simulink model "modele_gyros_BF1"  (Simulink 8.3)
settings: Solver=ode45  StartTime=0.0  StopTime=t_sim  RelTol=1e-3
values from neighbouring files (symbols this model uses):
  A = [0   0   0   0   1   0   0   0 ... (first row only)    [state_model_data.m]
  B = [0   0   0   0 ... (first row only)    [state_model_data.m]
  C = eye(8)    [state_model_data.m]
  Choix = 3    [script_axe3_BF.m]
  D = zeros(8, 4)    [state_model_data.m]
  Kg = 1/2*wn/zeta    (= 10.7142857143)    [script_axe3_BF.m]
  Kpv = 2*(Ic+Id)*wn*zeta    [script_axe3_BF.m]
  Omega1_0 = Omega1_c*2*pi/60    (= 41.8879020479)    [script_axe3_BF.m]
  Omega1_c = 400    [script_axe3_BF.m]
  Omega2_0 = 0    [script_axe3_BF.m]
  q20 = -pi/2    (= -1.57079632679)    [Traces_Gyros.m]    (also in script_axe3_BF.m = 0; state_model_data.m = 0)
  q30 = -pi/2    (= -1.57079632679)    [Traces_Gyros.m]    (also in script_axe3_BF.m = 0; state_model_data.m = 0)
undefined symbols (not defined in the file or in its folder): K1, K2, K3, K4, Kamp, Km1, Km2, Kv2, Kv3, Kv4, Omega2_c, Omega3_c, Omega4_c
libraries: library_gyro x1
settings Model: Creator=ahmed.chaibet  LastModifiedBy=ahmed.chaibet
settings OptimizationCC: ExpressionDepthLimit=2147483647
settings DebuggingCC: SaveWithParameterizedLinksMsg=none  SignalResolutionControl=TryResolveAllWithWarning  SolverPrmCheckMsg=none  MultiTaskDSMMsg=warning  MultiTaskCondExecSysMsg=none  StrictBusMsg=None
settings HardwareCC: TargetUnknown=on
settings RTWCC: IncludeERTFirstTime=on

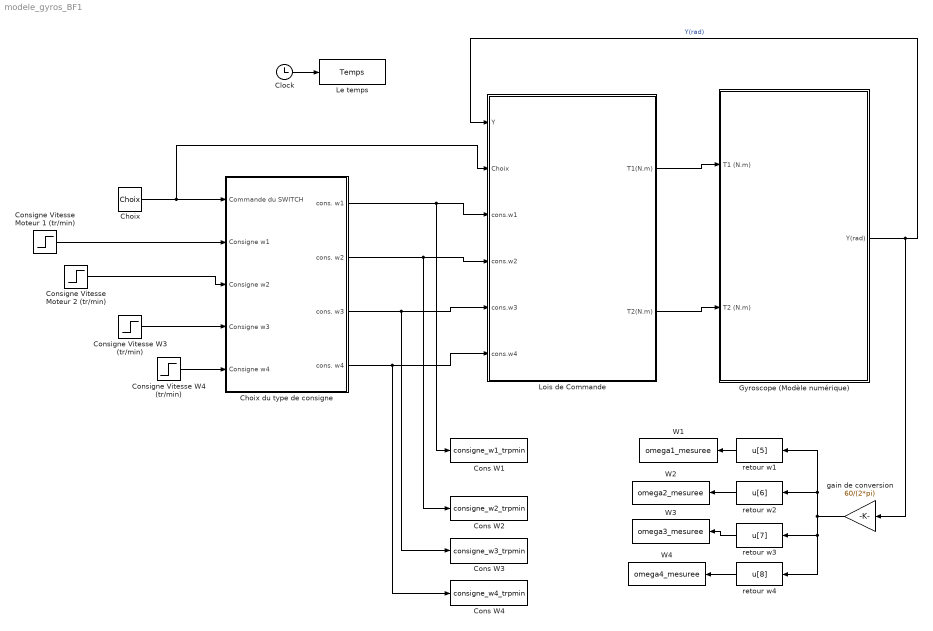
== system modele_gyros_BF1 ==
  Choix : Constant  Value=Choix
  Choix du type de consigne : Subsystem
  Clock : Clock
  Cons W1 : ToWorkspace  VariableName=consigne_w1_trpmin  SampleTime=-1
  Cons W2 : ToWorkspace  VariableName=consigne_w2_trpmin  SampleTime=-1
  Cons W3 : ToWorkspace  VariableName=consigne_w3_trpmin  SampleTime=-1
  Cons W4 : ToWorkspace  VariableName=consigne_w4_trpmin  SampleTime=-1
  Consigne Vitesse Moteur 1 (tr/min) : Step  Time=0  After=Omega1_c  SampleTime=0
  Consigne Vitesse Moteur 2 (tr/min) : Step  Time=0  After=Omega2_c  SampleTime=0
  Consigne Vitesse W3 (tr/min) : Step  Time=0  After=Omega3_c  SampleTime=0
  Consigne Vitesse W4 (tr/min) : Step  Time=0  After=Omega4_c  SampleTime=0
  Gyroscope (Modèle numérique) : Subsystem
  Le temps : ToWorkspace  VariableName=Temps  SampleTime=-1
  Lois de Commande : Subsystem
  W1 : ToWorkspace  VariableName=omega1_mesuree  SampleTime=-1
  W2 : ToWorkspace  VariableName=omega2_mesuree  SampleTime=-1
  W3 : ToWorkspace  VariableName=omega3_mesuree  SampleTime=-1
  W4 : ToWorkspace  VariableName=omega4_mesuree  SampleTime=-1
  gain de conversion : Gain  Gain=60/(2*pi)  SaturateOnIntegerOverflow=on  OutDataTypeStr=Inherit: Same as input  ParamDataTypeStr=Inherit: Same as input
  retour w1 : Fcn  Expr=u[5]
  retour w2 : Fcn  Expr=u[6]
  retour w3 : Fcn  Expr=u[7]
  retour w4 : Fcn  Expr=u[8]
  wires:
  Clock/1 -> Le temps/1
  Consigne Vitesse Moteur 1 (tr/min)/1 -> Choix du type de consigne/2(Consigne w1)
  Consigne Vitesse Moteur 2 (tr/min)/1 -> Choix du type de consigne/3(Consigne w2)
  Consigne Vitesse W3 (tr/min)/1 -> Choix du type de consigne/4(Consigne w3)
  Choix du type de consigne/1(cons. w1) -> Cons W1/1, Lois de Commande/3(cons.w1)
  Choix du type de consigne/2(cons. w2) -> Cons W2/1, Lois de Commande/4(cons.w2)
  Choix du type de consigne/3(cons. w3) -> Cons W3/1, Lois de Commande/5(cons.w3)
  Choix du type de consigne/4(cons. w4) -> Cons W4/1, Lois de Commande/6(cons.w4)
  Choix/1 -> Lois de Commande/2(Choix), Choix du type de consigne/1(Commande du SWITCH)
  Lois de Commande/1(T1(N.m)) -> Gyroscope (Modèle numérique)/1(T1 (N.m))
  Lois de Commande/2(T2(N.m)) -> Gyroscope (Modèle numérique)/2(T2 (N.m))
  Consigne Vitesse W4 (tr/min)/1 -> Choix du type de consigne/5(Consigne w4)
  Gyroscope (Modèle numérique)/1(Y(rad)) -> gain de conversion/1, Lois de Commande/1(Y)  "Y(rad)"
  gain de conversion/1 -> retour w1/1, retour w2/1, retour w4/1, retour w3/1
  retour w1/1 -> W1/1
  retour w2/1 -> W2/1
  retour w3/1 -> W3/1
  retour w4/1 -> W4/1

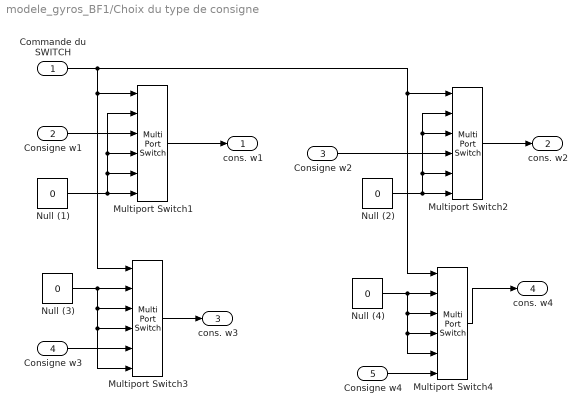
== system modele_gyros_BF1/Choix du type de consigne ==
  Commande du SWITCH : Inport
  Consigne w1 : Inport  Port=2
  Consigne w2 : Inport  Port=3
  Consigne w3 : Inport  Port=4
  Consigne w4 : Inport  Port=5
  Multiport Switch1 : MultiPortSwitch  Inputs=5  SaturateOnIntegerOverflow=on  InputSameDT=on
  Multiport Switch2 : MultiPortSwitch  Inputs=5  SaturateOnIntegerOverflow=on  InputSameDT=on
  Multiport Switch3 : MultiPortSwitch  Inputs=5  SaturateOnIntegerOverflow=on  InputSameDT=on
  "Multiport Switch4 " : MultiPortSwitch  Inputs=5  SaturateOnIntegerOverflow=on  InputSameDT=on
  Null (1) : Constant  Value=0
  Null (2) : Constant  Value=0
  Null (3) : Constant  Value=0
  Null (4) : Constant  Value=0
  cons. w1 : Outport
  cons. w2 : Outport  Port=2
  cons. w3 : Outport  Port=3
  cons. w4 : Outport  Port=4
  wires:
  Multiport Switch1/1 -> cons. w1/1
  Multiport Switch3/1 -> cons. w3/1
  Multiport Switch2/1 -> cons. w2/1
  "Multiport Switch4 "/1 -> cons. w4/1
  Commande du SWITCH/1 -> Multiport Switch1/1, Multiport Switch3/1, Multiport Switch2/1, "Multiport Switch4 "/1
  Consigne w1/1 -> Multiport Switch1/3
  Consigne w2/1 -> Multiport Switch2/4
  Consigne w3/1 -> Multiport Switch3/5
  Consigne w4/1 -> "Multiport Switch4 "/6
  Null (1)/1 -> Multiport Switch1/6, Multiport Switch1/5, Multiport Switch1/4, Multiport Switch1/2
  Null (2)/1 -> Multiport Switch2/6, Multiport Switch2/2, Multiport Switch2/3, Multiport Switch2/5
  Null (3)/1 -> Multiport Switch3/2, Multiport Switch3/3, Multiport Switch3/4, Multiport Switch3/6
  Null (4)/1 -> "Multiport Switch4 "/2, "Multiport Switch4 "/3, "Multiport Switch4 "/4, "Multiport Switch4 "/5

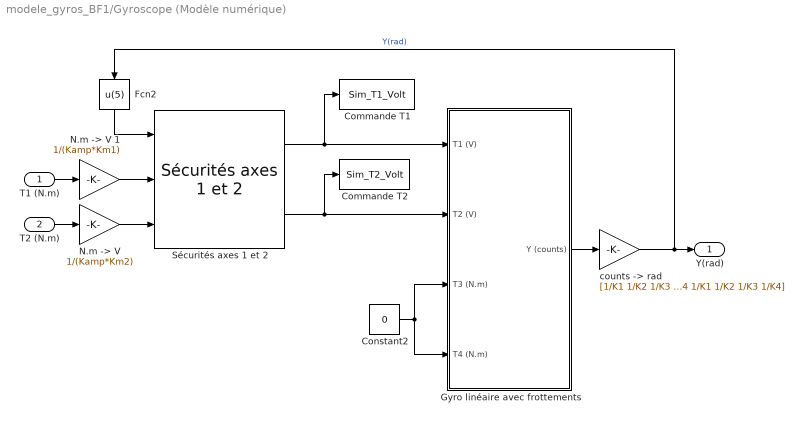
== system modele_gyros_BF1/Gyroscope (Modèle numérique) ==
  T1 (N.m) : Inport
  T2 (N.m) : Inport  Port=2
  Commande T1 : ToWorkspace  VariableName=Sim_T1_Volt  SampleTime=-1
  Commande T2 : ToWorkspace  VariableName=Sim_T2_Volt  SampleTime=-1
  Constant2 : Constant  Value=0
  Fcn2 : Fcn  Expr=u(5)
  Gyro linéaire avec frottements : Subsystem
  "N.m -> V" : Gain  Gain=1/(Kamp*Km2)  SaturateOnIntegerOverflow=on  OutDataTypeStr=Inherit: Same as input  ParamDataTypeStr=Inherit: Same as input
  "N.m -> V 1" : Gain  Gain=1/(Kamp*Km1)  SaturateOnIntegerOverflow=on  OutDataTypeStr=Inherit: Same as input  ParamDataTypeStr=Inherit: Same as input
  Sécurités axes 1 et 2 : library_gyro/Sécurités axes 1 et 2
  "counts -> rad" : Gain  Gain=[1/K1 1/K2 1/K3 1/K4 1/K1 1/K2 1/K3 1/K4]  SaturateOnIntegerOverflow=on  OutDataTypeStr=Inherit: Same as input  ParamDataTypeStr=Inherit: Same as input
  Y(rad) : Outport
  wires:
  Gyro linéaire avec frottements/1(Y (counts)) -> "counts -> rad"/1
  Sécurités axes 1 et 2/2 -> Gyro linéaire avec frottements/2(T2 (V)), Commande T2/1
  Sécurités axes 1 et 2/1 -> Gyro linéaire avec frottements/1(T1 (V)), Commande T1/1
  Constant2/1 -> Gyro linéaire avec frottements/4(T4 (N.m)), Gyro linéaire avec frottements/3(T3 (N.m))
  "N.m -> V"/1 -> Sécurités axes 1 et 2/3
  "counts -> rad"/1 -> Y(rad)/1, Fcn2/1  "Y(rad)"
  Fcn2/1 -> Sécurités axes 1 et 2/1
  "N.m -> V 1"/1 -> Sécurités axes 1 et 2/2
  T1 (N.m)/1 -> "N.m -> V 1"/1
  T2 (N.m)/1 -> "N.m -> V"/1

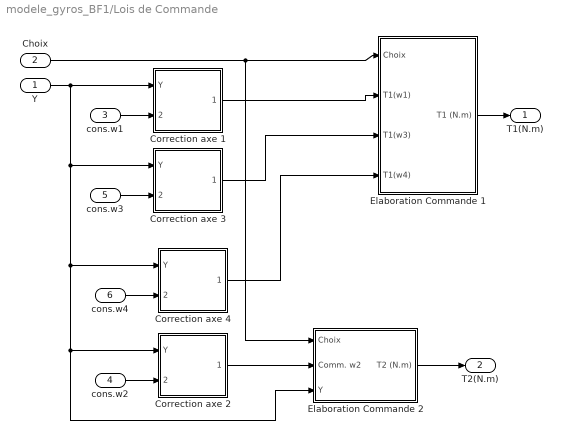
== system modele_gyros_BF1/Lois de Commande ==
  Y : Inport
  Choix : Inport  Port=2
  cons.w1 : Inport  Port=3
  cons.w2 : Inport  Port=4
  cons.w3 : Inport  Port=5
  cons.w4 : Inport  Port=6
  Correction axe 1 : Subsystem
  Correction axe 2 : Subsystem
  Correction axe 3 : Subsystem
  Correction axe 4 : Subsystem
  Elaboration Commande 1 : Subsystem
  Elaboration Commande 2 : Subsystem
  T1(N.m) : Outport
  T2(N.m) : Outport  Port=2
  wires:
  cons.w1/1 -> Correction axe 1/2(cons.w1)
  Correction axe 1/1(T1(w1)) -> Elaboration Commande 1/2(T1(w1))
  cons.w3/1 -> Correction axe 3/2(cons.w3)
  Correction axe 3/1(T1(w3)) -> Elaboration Commande 1/3(T1(w3))
  cons.w4/1 -> Correction axe 4/2(cons.w4)
  Correction axe 4/1(T2(w4)) -> Elaboration Commande 1/4(T1(w4))
  cons.w2/1 -> Correction axe 2/2(cons.w2)
  Correction axe 2/1(T2(w2)) -> Elaboration Commande 2/2(Comm. w2)
  Y/1 -> Correction axe 1/1(Y), Correction axe 3/1(Y), Correction axe 4/1(Y), Correction axe 2/1(Y), Elaboration Commande 2/3(Y)
  Elaboration Commande 1/1(T1 (N.m)) -> T1(N.m)/1
  Choix/1 -> Elaboration Commande 2/1(Choix), Elaboration Commande 1/1(Choix)
  Elaboration Commande 2/1(T2 (N.m)) -> T2(N.m)/1

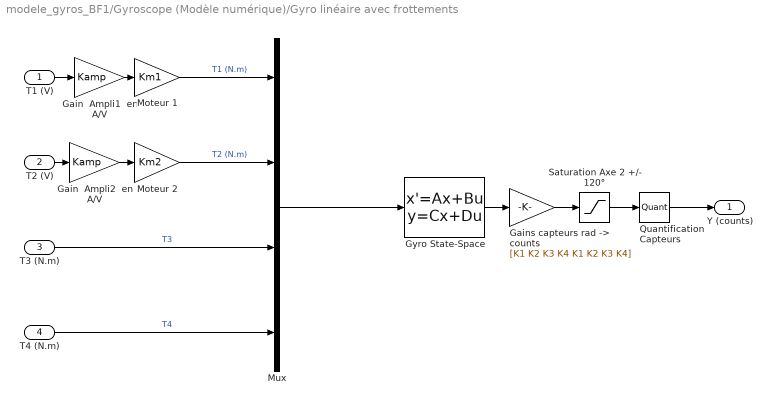
== system modele_gyros_BF1/Gyroscope (Modèle numérique)/Gyro linéaire avec frottements ==
  T1 (V) : Inport
  T2 (V) : Inport  Port=2
  T3 (N.m) : Inport  Port=3
  T4 (N.m) : Inport  Port=4
  Gain  Ampli1  en A/V : Gain  Gain=Kamp  SaturateOnIntegerOverflow=on  OutDataTypeStr=Inherit: Same as input  ParamDataTypeStr=Inherit: Same as input
  Gain  Ampli2  en A/V : Gain  Gain=Kamp  SaturateOnIntegerOverflow=on  OutDataTypeStr=Inherit: Same as input  ParamDataTypeStr=Inherit: Same as input
  "Gains capteurs rad -> counts" : Gain  Gain=[K1 K2 K3 K4 K1 K2 K3 K4]  SaturateOnIntegerOverflow=on  OutDataTypeStr=Inherit: Same as input  ParamDataTypeStr=Inherit: Same as input
  Gyro State-Space : StateSpace  A=A  B=B  C=C  D=D  X0=[0 q20 q30 0 Omega1_0 Omega2_0 0 0]
  Moteur 1 : Gain  Gain=Km1  SaturateOnIntegerOverflow=on  OutDataTypeStr=Inherit: Same as input  ParamDataTypeStr=Inherit: Same as input
  Moteur 2 : Gain  Gain=Km2  SaturateOnIntegerOverflow=on  OutDataTypeStr=Inherit: Same as input  ParamDataTypeStr=Inherit: Same as input
  Mux : Mux
  Quantification Capteurs : Quantizer  QuantizationInterval=Q
  Saturation Axe 2 +/- 120° : Saturate  UpperLimit=[inf 120*pi/180*K2 inf inf inf inf inf inf]  LowerLimit=[-inf -120*pi/180*K2 -inf -inf -inf -inf -inf -inf]
  Y (counts) : Outport
  wires:
  T1 (V)/1 -> Gain  Ampli1  en A/V/1
  Gain  Ampli1  en A/V/1 -> Moteur 1/1
  Moteur 2/1 -> Mux/2  "T2 (N.m)"
  Gain  Ampli2  en A/V/1 -> Moteur 2/1
  Gyro State-Space/1 -> "Gains capteurs rad -> counts"/1
  T2 (V)/1 -> Gain  Ampli2  en A/V/1
  Saturation Axe 2 +/- 120°/1 -> Quantification Capteurs/1
  Quantification Capteurs/1 -> Y (counts)/1
  T3 (N.m)/1 -> Mux/3  "T3"
  T4 (N.m)/1 -> Mux/4  "T4"
  "Gains capteurs rad -> counts"/1 -> Saturation Axe 2 +/- 120°/1
  Moteur 1/1 -> Mux/1  "T1 (N.m)"
  Mux/1 -> Gyro State-Space/1

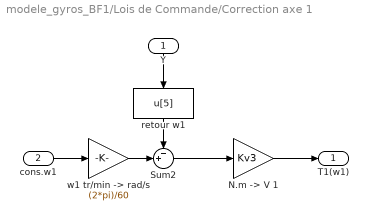
== system modele_gyros_BF1/Lois de Commande/Correction axe 1 ==
  Y : Inport
  cons.w1 : Inport  Port=2
  "N.m -> V 1" : Gain  Gain=Kv3  SaturateOnIntegerOverflow=on  OutDataTypeStr=Inherit: Same as input  ParamDataTypeStr=Inherit: Same as input
  Sum2 : Sum  Inputs=-+|  SaturateOnIntegerOverflow=on  InputSameDT=on  OutDataTypeStr=Inherit: Same as first input
  retour w1 : Fcn  Expr=u[5]
  "w1 tr/min -> rad/s" : Gain  Gain=(2*pi)/60  SaturateOnIntegerOverflow=on  OutDataTypeStr=Inherit: Same as input  ParamDataTypeStr=Inherit: Same as input
  T1(w1) : Outport
  wires:
  "w1 tr/min -> rad/s"/1 -> Sum2/2
  retour w1/1 -> Sum2/1
  Sum2/1 -> "N.m -> V 1"/1
  cons.w1/1 -> "w1 tr/min -> rad/s"/1
  "N.m -> V 1"/1 -> T1(w1)/1
  Y/1 -> retour w1/1

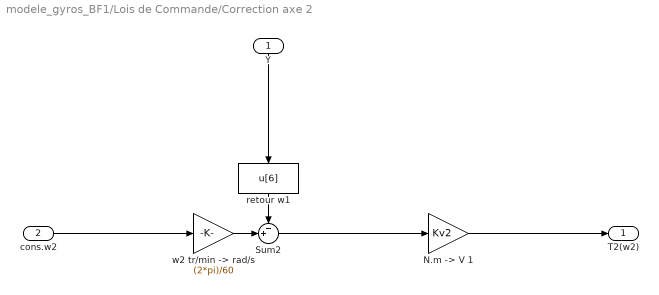
== system modele_gyros_BF1/Lois de Commande/Correction axe 2 ==
  Y : Inport
  cons.w2 : Inport  Port=2
  "N.m -> V 1" : Gain  Gain=Kv2  SaturateOnIntegerOverflow=on  OutDataTypeStr=Inherit: Same as input  ParamDataTypeStr=Inherit: Same as input
  Sum2 : Sum  Inputs=-+|  SaturateOnIntegerOverflow=on  InputSameDT=on  OutDataTypeStr=Inherit: Same as first input
  retour w1 : Fcn  Expr=u[6]
  "w2 tr/min -> rad/s" : Gain  Gain=(2*pi)/60  SaturateOnIntegerOverflow=on  OutDataTypeStr=Inherit: Same as input  ParamDataTypeStr=Inherit: Same as input
  T2(w2) : Outport
  wires:
  "w2 tr/min -> rad/s"/1 -> Sum2/2
  retour w1/1 -> Sum2/1
  Sum2/1 -> "N.m -> V 1"/1
  cons.w2/1 -> "w2 tr/min -> rad/s"/1
  "N.m -> V 1"/1 -> T2(w2)/1
  Y/1 -> retour w1/1

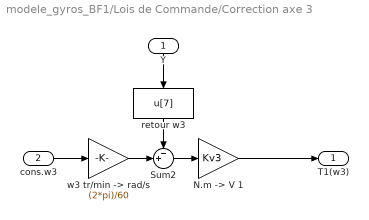
== system modele_gyros_BF1/Lois de Commande/Correction axe 3 ==
  Y : Inport
  cons.w3 : Inport  Port=2
  "N.m -> V 1" : Gain  Gain=Kv3  SaturateOnIntegerOverflow=on  OutDataTypeStr=Inherit: Same as input  ParamDataTypeStr=Inherit: Same as input
  Sum2 : Sum  Inputs=-+|  SaturateOnIntegerOverflow=on  InputSameDT=on  OutDataTypeStr=Inherit: Same as first input
  retour w3 : Fcn  Expr=u[7]
  "w3 tr/min -> rad/s" : Gain  Gain=(2*pi)/60  SaturateOnIntegerOverflow=on  OutDataTypeStr=Inherit: Same as input  ParamDataTypeStr=Inherit: Same as input
  T1(w3) : Outport
  wires:
  Y/1 -> retour w3/1
  "N.m -> V 1"/1 -> T1(w3)/1
  cons.w3/1 -> "w3 tr/min -> rad/s"/1
  Sum2/1 -> "N.m -> V 1"/1
  retour w3/1 -> Sum2/1
  "w3 tr/min -> rad/s"/1 -> Sum2/2

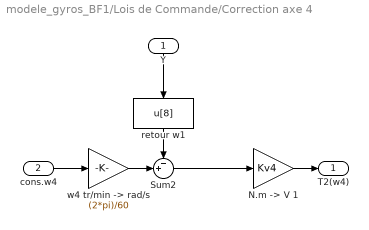
== system modele_gyros_BF1/Lois de Commande/Correction axe 4 ==
  Y : Inport
  cons.w4 : Inport  Port=2
  "N.m -> V 1" : Gain  Gain=Kv4  SaturateOnIntegerOverflow=on  OutDataTypeStr=Inherit: Same as input  ParamDataTypeStr=Inherit: Same as input
  Sum2 : Sum  Inputs=-+|  SaturateOnIntegerOverflow=on  InputSameDT=on  OutDataTypeStr=Inherit: Same as first input
  retour w1 : Fcn  Expr=u[8]
  "w4 tr/min -> rad/s" : Gain  Gain=(2*pi)/60  SaturateOnIntegerOverflow=on  OutDataTypeStr=Inherit: Same as input  ParamDataTypeStr=Inherit: Same as input
  T2(w4) : Outport
  wires:
  Y/1 -> retour w1/1
  "N.m -> V 1"/1 -> T2(w4)/1
  cons.w4/1 -> "w4 tr/min -> rad/s"/1
  Sum2/1 -> "N.m -> V 1"/1
  retour w1/1 -> Sum2/1
  "w4 tr/min -> rad/s"/1 -> Sum2/2

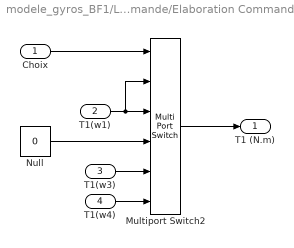
== system modele_gyros_BF1/Lois de Commande/Elaboration Commande 1 ==
  Choix : Inport
  T1(w1) : Inport  Port=2
  T1(w3) : Inport  Port=3
  T1(w4) : Inport  Port=4
  Multiport Switch2 : MultiPortSwitch  Inputs=5  SaturateOnIntegerOverflow=on  InputSameDT=on
  Null : Constant  Value=0
  T1 (N.m) : Outport
  wires:
  Choix/1 -> Multiport Switch2/1
  T1(w1)/1 -> Multiport Switch2/3, Multiport Switch2/2
  Multiport Switch2/1 -> T1 (N.m)/1
  T1(w3)/1 -> Multiport Switch2/5
  Null/1 -> Multiport Switch2/4
  T1(w4)/1 -> Multiport Switch2/6

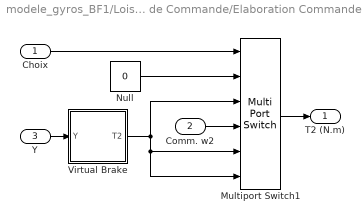
== system modele_gyros_BF1/Lois de Commande/Elaboration Commande 2 ==
  Choix : Inport
  Comm. w2 : Inport  Port=2
  Y : Inport  Port=3
  Multiport Switch1 : MultiPortSwitch  Inputs=5  SaturateOnIntegerOverflow=on  InputSameDT=on
  Null : Constant  Value=0
  Virtual Brake : Subsystem
  T2 (N.m) : Outport
  wires:
  Choix/1 -> Multiport Switch1/1
  Multiport Switch1/1 -> T2 (N.m)/1
  Y/1 -> Virtual Brake/1(Y)
  Null/1 -> Multiport Switch1/2
  Virtual Brake/1(T2) -> Multiport Switch1/3, Multiport Switch1/5, Multiport Switch1/6
  Comm. w2/1 -> Multiport Switch1/4

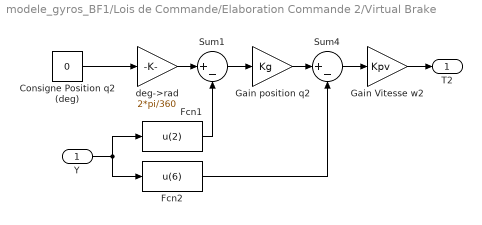
== system modele_gyros_BF1/Lois de Commande/Elaboration Commande 2/Virtual Brake ==
  Y : Inport
  Consigne Position q2 (deg) : Constant  Value=0
  Fcn1 : Fcn  Expr=u(2)
  Fcn2 : Fcn  Expr=u(6)
  Gain Vitesse w2 : Gain  Gain=Kpv  SaturateOnIntegerOverflow=on  OutDataTypeStr=Inherit: Same as input  ParamDataTypeStr=Inherit: Same as input
  Gain position q2 : Gain  Gain=Kg  SaturateOnIntegerOverflow=on  OutDataTypeStr=Inherit: Same as input  ParamDataTypeStr=Inherit: Same as input
  Sum1 : Sum  Inputs=|+-  SaturateOnIntegerOverflow=on  InputSameDT=on  OutDataTypeStr=Inherit: Same as first input
  Sum4 : Sum  Inputs=|+-  SaturateOnIntegerOverflow=on  InputSameDT=on  OutDataTypeStr=Inherit: Same as first input
  deg->rad : Gain  Gain=2*pi/360  SaturateOnIntegerOverflow=on  OutDataTypeStr=Inherit: Same as input  ParamDataTypeStr=Inherit: Same as input
  T2 : Outport
  wires:
  Fcn1/1 -> Sum1/2
  Sum1/1 -> Gain position q2/1
  Sum4/1 -> Gain Vitesse w2/1
  Fcn2/1 -> Sum4/2
  Consigne Position q2 (deg)/1 -> deg->rad/1
  Gain position q2/1 -> Sum4/1
  Y/1 -> Fcn2/1, Fcn1/1
  Gain Vitesse w2/1 -> T2/1
  deg->rad/1 -> Sum1/1
